simulink model "mechanicalsystem"  (R2024b)
settings: Solver=VariableStepAuto  StartTime=0.0  StopTime=10.0  RelTol=1e-3

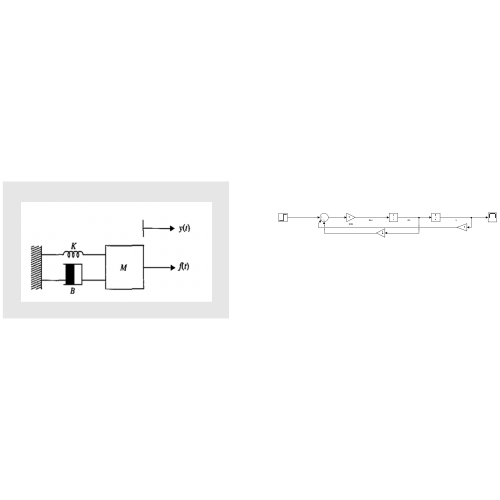
[thumbnail: Simulink's stored preview of the top-level diagram]
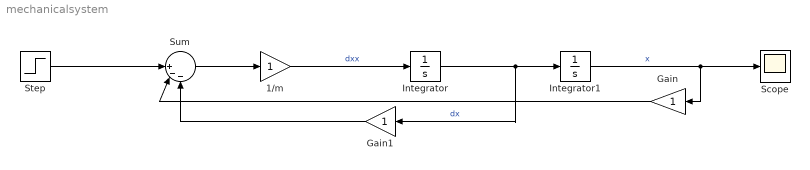
== system mechanicalsystem ==
  1/m : Gain
  Gain : Gain
  Gain1 : Gain
  Integrator : Integrator
  Integrator1 : Integrator  ContinuousStateAttributes=x
  Scope : Scope
  Step : Step  SampleTime=0
  Sum : Sum  Inputs=||+--
  wires:
  Integrator/1 -> Gain1/1, Integrator1/1  "dx"
  Integrator1/1 -> Scope/1, Gain/1  "x"
  Gain/1 -> Sum/2
  Gain1/1 -> Sum/3
  Sum/1 -> 1/m/1
  1/m/1 -> Integrator/1  "dxx"
  Step/1 -> Sum/1
